simulink model "old_model_new"  (R2023a)
settings: Solver=VariableStepAuto  StartTime=0.0  StopTime=1  RelTol=1e-3
undefined symbols (not defined in the file or in its folder): Ts
libraries: simulink x6, spsVoltageMeasurementLib x3, spsDCVoltageSourceLib x1, slpidlib x1, spsTriangleGeneratorLib x1, spsPermanentMagnetSynchronousMachineLib x1, spsUniversalBridgeLib x1, spspowerguiLib x1
settings Model: Creator=ahmedmajid  LastModifiedBy=ahmedmajid
settings RTWCC: GPUComputeCapability=5.0

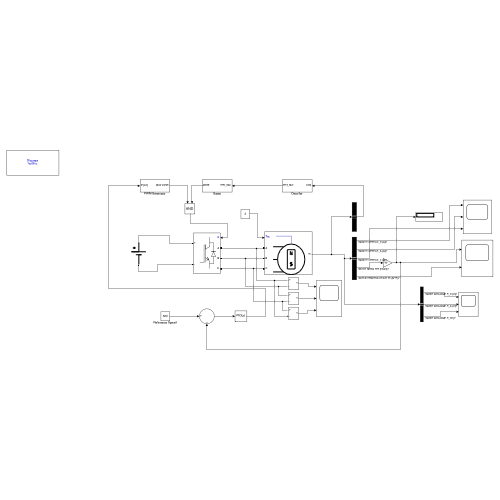
[thumbnail: Simulink's stored preview of the top-level diagram]
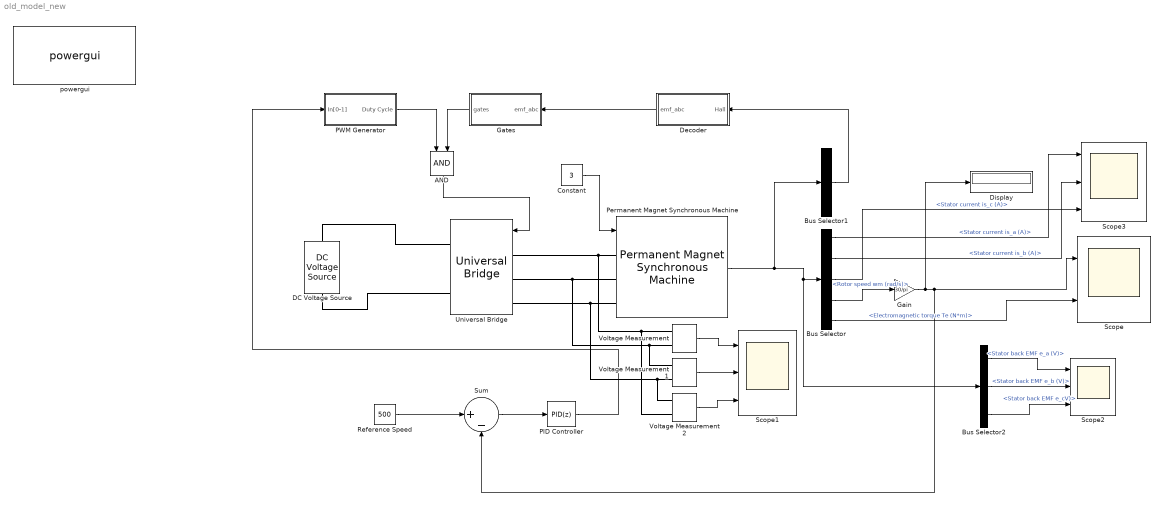
== system old_model_new ==
  AND : Logic  AllPortsSameDT=off  OutDataTypeStr=boolean
  Bus Selector : BusSelector  OutputSignals=Stator current is_a (A),Stator current is_b (A),Stator current is_c (A),Rotor speed wm (rad/s),Electromagnetic torque Te (N*m)
  Bus Selector1 : BusSelector  OutputSignals=Hall effect signal h_a,Hall effect signal h_b,Hall effect signal h_c  OutputAsBus=on
  Bus Selector2 : BusSelector  OutputSignals=Stator back EMF e_a (V),Stator back EMF e_b (V),Stator back EMF e_cV)
  Constant : Constant  Value=3
  DC Voltage Source : spsDCVoltageSourceLib/DC Voltage Source  Amplitude=400  Measurements=None
  Decoder : Subsystem
  Display : Display
  Gain : Gain  Gain=30/pi
  Gates : Subsystem
  PID Controller : slpidlib/PID Controller  Controller=PID  Form=Parallel  TimeDomain=Discrete-time  UseExternalTs=off  SampleTime=-1  IntegratorMethod=Forward Euler  FilterMethod=Forward Euler  ControllerParametersSource=internal  P=2  I=1  UseKiTs=off  D=.01  N=100  UseFilter=on  TunerSelectOption=Transfer Function Based (PID Tuner App)  InitialConditionSource=internal  InitialConditionForIntegrator=0  InitialConditionForFilter=0  DifferentiatorICPrevScaledInput=0  ExternalReset=none  TrackingMode=off  Kt=1  LimitOutput=off  SatLimitsSource=internal  UpperSaturationLimit=inf  LowerSaturationLimit=-inf  LinearizeAsGain=on  AntiWindupMode=none  Kb=1  LimitIntegrator=off  UpperIntegratorSaturationLimit=inf  LowerIntegratorSaturationLimit=-inf  POutMin=[]  POutMax=[]  IOutMin=[]  IOutMax=[]  DOutMin=[]  DOutMax=[]  NOutMin=[]  NOutMax=[]  SumOutMin=[]  SumOutMax=[]  SaturationOutMin=[]  SaturationOutMax=[]  PParamMin=[]  PParamMax=[]  IParamMin=[]  IParamMax=[]  DParamMin=[]  DParamMax=[]  NParamMin=[]  NParamMax=[]  KbParamMin=[]  KbParamMax=[]  KtParamMin=[]  KtParamMax=[]  KbOutMin=[]  KbOutMax=[]  KtOutMin=[]  KtOutMax=[]  IntegratorOutMin=[]  IntegratorOutMax=[]  FilterOutMin=[]  FilterOutMax=[]  SumI1OutMin=[]  SumI1OutMax=[]  SumI2OutMin=[]  SumI2OutMax=[]  SumI3OutMin=[]  SumI3OutMax=[]  SumI4OutMin=[]  SumI4OutMax=[]  SumDOutMin=[]  SumDOutMax=[]  DifferentiatorOutMin=[]  DifferentiatorOutMax=[]  FilterDiffOutCoefMin=[]  FilterDiffOutCoefMax=[]  ReciprocalOutMin=[]  ReciprocalOutMax=[]  SumDenOutMin=[]  SumDenOutMax=[]  SumNumOutMin=[]  SumNumOutMax=[]  DivideOutMin=[]  DivideOutMax=[]  UdiffTsProdOutMin=[]  UdiffTsProdOutMax=[]  NTsProdOutMin=[]  NTsProdOutMax=[]  UintegralTsProdOutMin=[]  UintegralTsProdOutMax=[]  UngainTsProdOutMin=[]  UngainTsProdOutMax=[]  ClampingZeroOutDataTypeStr=Inherit: Inherit via back propagation  ClampingZeroOutMin=[]  ClampingZeroOutMax=[]  FilterDenConstantOutDataTypeStr=Inherit: Inherit via back propagation  FilterDenConstantOutMin=[]  FilterDenConstantOutMax=[]  PCopyOutDataTypeStr=Inherit: Inherit via back propagation  PCopyOutMin=[]  PCopyOutMax=[]  NCopyOutDataTypeStr=Inherit: Inherit via back propagation  NCopyOutMin=[]  NCopyOutMax=[]  IntegratorContinuousStateAttributes=''  IntegratorStateMustResolveToSignalObject=off  IntegratorRTWStateStorageClass=Auto  FilterContinuousStateAttributes=''  FilterStateMustResolveToSignalObject=off  FilterRTWStateStorageClass=Auto  ParallelPVariant=InternalParameters  IdealPVariant=Disabled  IVariant=InternalParameters  DVariant=InternalParameters  IntegratorVariant=Discrete  SatVariant=Disabled  AWVariant=Passthrough  PCopyVariant=Disabled  TRVariant=Disabled  FdbkBlocksVariant=Forward  IdealPFdbkVariant=Disabled  SatFdbkVariant=Disabled  DerivativeFilterVariant=ForwardEulerFilter  NVariant=InternalParameters  NCopyVariant=Disabled  FilterICVariant=InternalICsFilter  IntegratorICVariant=InternalICs  ExternalResetVariant=Disabled  TRSumVariant=Passthrough  SumFdbkVariant=Disabled  SumVariant=Sum_PID  TsampFilterVariant=InternalTs  TsampNgainVariant=Passthrough  TsampIntegralVariant=Disabled_SignalSpec  ExternalSaturationOutDataTypeStr=Inherit: Same as second input
  PWM Generator : Subsystem
  Permanent Magnet Synchronous Machine : spsPermanentMagnetSynchronousMachineLib/Permanent Magnet Synchronous Machine  NbPhases=3  FluxDistribution=Trapezoidal  RotorType=Round  MechanicalLoad=Torque Tm  PresetModel="01:  0.8 Nm 300 Vdc 3000 RPM - 0.8 Nm"  ShowDetailedParameters=on  MeasurementBus=off  Resistance=0.007  Inductance=0.0003  dqInductances=[8.5e-3,8.5e-3]  La=0.02682  MachineConstant=Flux linkage established by magnets (V.s)  Flux=0.1716  VoltageCst=71.8796  TorqueCst=0.6864  Flat=120  Mechanical=[2.26e-05 1.349e-05 2 0]  PolePairs=2  InitialConditions=[0,0, 0,0]  InitialConditions5ph=[0 0 0 0 0 0]  RefAngle=Aligned with phase A axis (original Park)  IterativeDiscreteModel=Trapezoidal robust  TsBlock=1e-5  TsPowergui=0
  Reference Speed : Constant  Value=500
  Scope : Scope  NumInputPorts=2
  Scope1 : Scope  NumInputPorts=3
  Scope2 : Scope  NumInputPorts=3
  Scope3 : Scope  NumInputPorts=3
  Sum : Sum  Inputs=|+-
  Universal Bridge : spsUniversalBridgeLib/Universal Bridge  Arms=3  SnubberResistance=1e5  SnubberCapacitance=inf  Device=IGBT / Diodes  Ron=1e-3  Lon=0  ForwardVoltages="[  0  0  ]"  ForwardVoltage=0  GTOparameters=[ 10e-6 , 20e-6 ]  IGBTparameters=[ 1e-6 , 2e-6 ]  Measurements=None  Measurements_2=None  converterType=Rectifier
  Voltage Measurement : spsVoltageMeasurementLib/Voltage Measurement  PhasorSimulation=off  OutputType=Complex  PSBequivalent=0
  Voltage Measurement1 : spsVoltageMeasurementLib/Voltage Measurement  PhasorSimulation=off  OutputType=Complex  PSBequivalent=0
  Voltage Measurement2 : spsVoltageMeasurementLib/Voltage Measurement  PhasorSimulation=off  OutputType=Complex  PSBequivalent=0
  powergui : spspowerguiLib/powergui  Priority=1  SimulationMode=Discrete  SampleTime=Ts  frequency=60  Iterations=50  frequencyindice=0  Pbase=100e6  ErrMax=1e-4  UnitsV=kV  UnitsW=MW  buscounter=0  FunctionMessages=off  echomessages=off  EnableUseOfTLC=off  CurrentSourceSwitches=off  DisableSnubberDevices=off  DisableRonSwitches=off  DisableVfSwitches=off  DisplayEquations=off  AutomaticDiscreteSolvers=off  SolverType=Tustin/Backward Euler (TBE)  Interpol=off  ExternalGateDelay=off  methode=off  Ts=100  x0status=blocks  SPID=on  SwTol=0  HookPort=off  NonlinearTolerance=1e-4  nMaxIteration=100  ContinueOnMaxIteration=off  RestoreLinks=warning  ResistiveCurrentMeasurement=off  Frange=[0:2:500]  Ylog=off  Xlog=on  ShowGrid=off  save=off  variable=ZData  structure=0  ZoomFFT=off  StartTime=0.0  cycles=1  DisplayStyle=1  fundamental=60  FreqAxis=off  MaxFrequency=1000  frequencyindicesteady=1  RmsSteady=1  display=off
  wires:
  Reference Speed/1 -> Sum/1
  Sum/1 -> PID Controller/1
  Permanent Magnet Synchronous Machine/1 -> Bus Selector1/1, Bus Selector2/1, Bus Selector/1
  Gain/1 -> Scope/1, Sum/2, Display/1
  Bus Selector1/1 -> Decoder/1(Hall)
  Decoder/1(emf_abc) -> Gates/1(emf_abc)
  Gates/1(gates) -> AND/2
  PWM Generator/1(Duty Cycle) -> AND/1
  AND/1 -> Universal Bridge/1
  Constant/1 -> Permanent Magnet Synchronous Machine/1
  PID Controller/1 -> PWM Generator/1(In[0-1])
  Bus Selector2/1 -> Scope2/1  "<Stator back EMF e_a (V)>"
  Bus Selector2/2 -> Scope2/2  "<Stator back EMF e_b (V)>"
  Bus Selector2/3 -> Scope2/3  "<Stator back EMF e_cV)>"
  Bus Selector/1 -> Scope3/1  "<Stator current is_a (A)>"
  Bus Selector/2 -> Scope3/2  "<Stator current is_b (A)>"
  Bus Selector/3 -> Scope3/3  "<Stator current is_c (A)>"
  Bus Selector/4 -> Gain/1  "<Rotor speed wm (rad/s)>"
  Bus Selector/5 -> Scope/2  "<Electromagnetic torque Te (N*m)>"
  Voltage Measurement/1 -> Scope1/1
  Voltage Measurement1/1 -> Scope1/2
  Voltage Measurement2/1 -> Scope1/3
  connections:
  Universal Bridge/LConn1 -- Voltage Measurement2/LConn2 -- Voltage Measurement/LConn1 -- Permanent Magnet Synchronous Machine/LConn1
  Universal Bridge/LConn2 -- Voltage Measurement1/LConn1 -- Voltage Measurement/LConn2 -- Permanent Magnet Synchronous Machine/LConn2
  Permanent Magnet Synchronous Machine/LConn3 -- Voltage Measurement2/LConn1 -- Voltage Measurement1/LConn2 -- Universal Bridge/LConn3
  DC Voltage Source/RConn1 -- Universal Bridge/RConn1
  DC Voltage Source/LConn1 -- Universal Bridge/RConn2

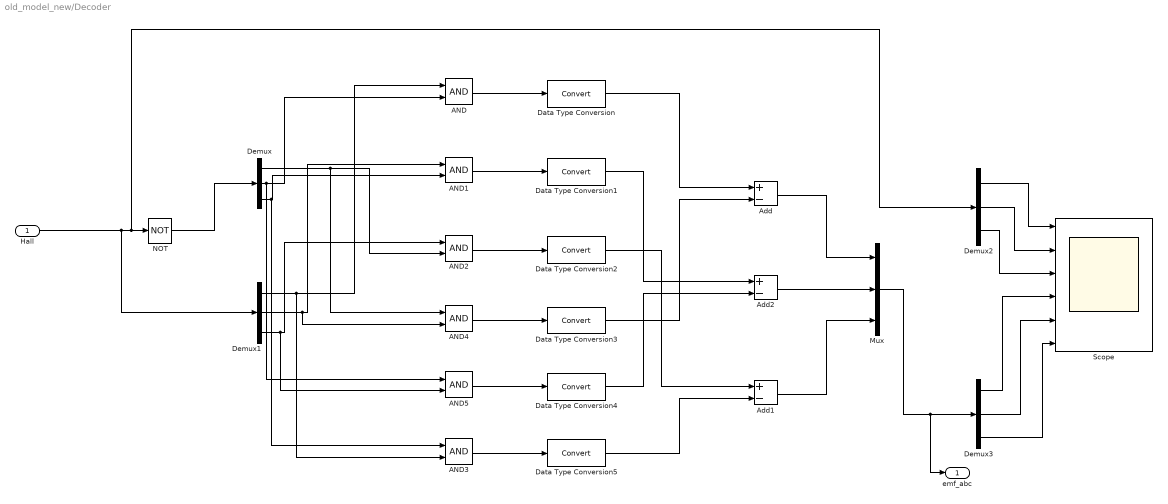
== system old_model_new/Decoder ==
  Hall : Inport
  AND{,1..5} (6 alike) : Logic  AllPortsSameDT=off  OutDataTypeStr=boolean
  Add : Sum  Inputs=+-
  Add1 : Sum  Inputs=+-
  Add2 : Sum  Inputs=+-
  Data Type Conversion{,1..5} (6 alike) : DataTypeConversion  SaturateOnIntegerOverflow=off  RndMeth=Floor
  Demux{,1..3} (4 alike) : Demux  Outputs=3
  Mux : Mux  Inputs=3
  NOT : Logic  Operator=NOT  AllPortsSameDT=off  OutDataTypeStr=boolean
  Scope : Scope  NumInputPorts=6
  emf_abc : Outport
  wires:
  Hall/1 -> Demux2/1, NOT/1, Demux1/1
  NOT/1 -> Demux/1
  Demux1/2 -> AND4/2, AND1/1
  Demux1/3 -> AND5/2, AND2/1
  Demux/2 -> AND5/1, AND/2
  Demux/3 -> AND3/1, AND1/2
  Demux/1 -> AND4/1, AND2/2
  Demux1/1 -> AND3/2, AND/1
  AND/1 -> Data Type Conversion/1
  AND1/1 -> Data Type Conversion1/1
  AND2/1 -> Data Type Conversion2/1
  AND4/1 -> Data Type Conversion3/1
  AND5/1 -> Data Type Conversion4/1
  AND3/1 -> Data Type Conversion5/1
  Data Type Conversion/1 -> Add/1
  Data Type Conversion3/1 -> Add/2
  Data Type Conversion1/1 -> Add2/1
  Data Type Conversion4/1 -> Add2/2
  Data Type Conversion2/1 -> Add1/1
  Data Type Conversion5/1 -> Add1/2
  Add2/1 -> Mux/2
  Add/1 -> Mux/1
  Add1/1 -> Mux/3
  Mux/1 -> emf_abc/1, Demux3/1
  Demux2/1 -> Scope/1
  Demux2/2 -> Scope/2
  Demux2/3 -> Scope/3
  Demux3/1 -> Scope/4
  Demux3/2 -> Scope/5
  Demux3/3 -> Scope/6

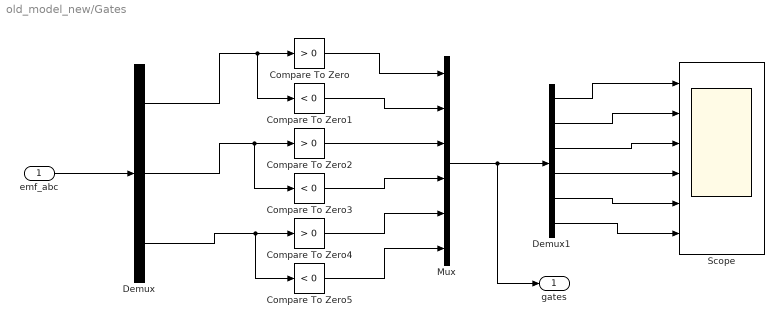
== system old_model_new/Gates ==
  emf_abc : Inport
  Compare To Zero : simulink/Logic and Bit Operations/Compare To Zero  relop=>  OutDataTypeStr=boolean
  Compare To Zero1 : simulink/Logic and Bit Operations/Compare To Zero  relop=<  OutDataTypeStr=boolean
  Compare To Zero2 : simulink/Logic and Bit Operations/Compare To Zero  relop=>  OutDataTypeStr=boolean
  Compare To Zero3 : simulink/Logic and Bit Operations/Compare To Zero  relop=<  OutDataTypeStr=boolean
  Compare To Zero4 : simulink/Logic and Bit Operations/Compare To Zero  relop=>  OutDataTypeStr=boolean
  Compare To Zero5 : simulink/Logic and Bit Operations/Compare To Zero  relop=<  OutDataTypeStr=boolean
  Demux : Demux  Outputs=3
  Demux1 : Demux  Outputs=6
  Mux : Mux  Inputs=6
  Scope : Scope  NumInputPorts=6
  gates : Outport
  wires:
  emf_abc/1 -> Demux/1
  Demux/1 -> Compare To Zero1/1, Compare To Zero/1
  Demux/2 -> Compare To Zero3/1, Compare To Zero2/1
  Demux/3 -> Compare To Zero5/1, Compare To Zero4/1
  Compare To Zero/1 -> Mux/1
  Compare To Zero1/1 -> Mux/2
  Compare To Zero2/1 -> Mux/3
  Compare To Zero3/1 -> Mux/4
  Compare To Zero4/1 -> Mux/5
  Compare To Zero5/1 -> Mux/6
  Mux/1 -> gates/1, Demux1/1
  Demux1/1 -> Scope/1
  Demux1/2 -> Scope/2
  Demux1/3 -> Scope/3
  Demux1/4 -> Scope/4
  Demux1/5 -> Scope/5
  Demux1/6 -> Scope/6

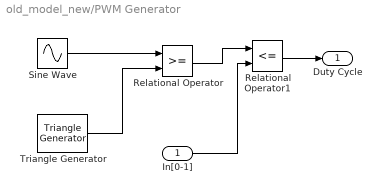
== system old_model_new/PWM Generator ==
  In[0-1] : Inport
  Relational Operator : RelationalOperator  OutDataTypeStr=boolean  RndMeth=Simplest  InputSameDT=off
  Relational Operator1 : RelationalOperator  Operator=<=  OutDataTypeStr=boolean  RndMeth=Simplest  InputSameDT=off
  Sine Wave : Sin  Frequency=2*pi*50  SampleTime=0
  Triangle Generator : spsTriangleGeneratorLib/Triangle Generator  Freq=10e3  Phase=0  Ts=0
  Duty Cycle : Outport
  wires:
  Sine Wave/1 -> Relational Operator/1
  Triangle Generator/1 -> Relational Operator/2
  Relational Operator/1 -> Relational Operator1/1
  In[0-1]/1 -> Relational Operator1/2
  Relational Operator1/1 -> Duty Cycle/1
